simulink model "part3_3_b"  (R2017b)
settings: Solver=VariableStepAuto  StartTime=0.0  StopTime=0.1  RelTol=1e-3
libraries: simulink x1
settings Model: Creator=think  LastModifiedBy=think

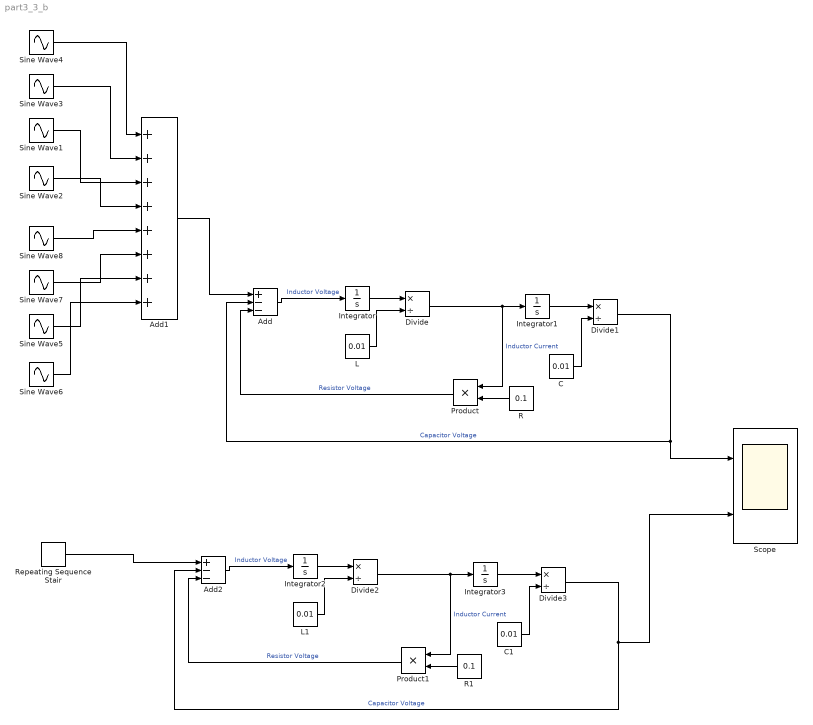
== system part3_3_b ==
  Add : Sum  Inputs=+--
  Add1 : Sum  Inputs=++++++++
  Add2 : Sum  Inputs=+--
  C : Constant  Value=0.01
  C1 : Constant  Value=0.01
  Divide{,1..3} (4 alike) : Product  Inputs=*/
  Integrator{,1..3} (4 alike) : Integrator
  L : Constant  Value=0.01
  L1 : Constant  Value=0.01
  Product : Product
  Product1 : Product
  R : Constant  Value=0.1
  R1 : Constant  Value=0.1
  Repeating Sequence Stair : simulink/Sources/Repeating Sequence Stair  OutValues=[1 -1]  tsamp=1/64  OutMin=[]  OutMax=[]  OutDataTypeStr=double  OutputDataTypeScalingMode=double  OutDataType=fixdt(0,8)  ConRadixGroup=Best Precision: Vector-wise  OutScaling=2^-12
  Scope : Scope  NumInputPorts=2
  Sine Wave1 : Sin  Amplitude=(4/pi)/5  Frequency=2*pi*32*5  SampleTime=0
  Sine Wave2 : Sin  Amplitude=(4/pi)/7  Frequency=2*pi*32*7  SampleTime=0
  Sine Wave3 : Sin  Amplitude=(4/pi)/3  Frequency=(2*pi*32)*3  SampleTime=0
  Sine Wave4 : Sin  Amplitude=4/pi  Frequency=2*pi*32  SampleTime=0
  Sine Wave5 : Sin  Amplitude=(4/pi)/13  Frequency=2*pi*32*13  SampleTime=0
  Sine Wave6 : Sin  Amplitude=(4/pi)/15  Frequency=2*pi*32*15  SampleTime=0
  Sine Wave7 : Sin  Amplitude=(4/pi)/11  Frequency=(2*pi*32)*11  SampleTime=0
  Sine Wave8 : Sin  Amplitude=4/pi/9  Frequency=2*pi*32*9  SampleTime=0
  wires:
  C/1 -> Divide1/2
  Integrator/1 -> Divide/1
  Integrator1/1 -> Divide1/1
  Divide/1 -> Integrator1/1, Product/1  "Inductor Current"
  Add/1 -> Integrator/1  "Inductor Voltage"
  Product/1 -> Add/3  "Resistor Voltage"
  L/1 -> Divide/2
  R/1 -> Product/2
  Divide1/1 -> Add/2, Scope/1  "Capacitor Voltage"
  Sine Wave2/1 -> Add1/4
  Sine Wave1/1 -> Add1/3
  Sine Wave4/1 -> Add1/1
  Sine Wave3/1 -> Add1/2
  Add1/1 -> Add/1
  Integrator3/1 -> Divide3/1
  Add2/1 -> Integrator2/1  "Inductor Voltage"
  Divide2/1 -> Integrator3/1, Product1/1  "Inductor Current"
  C1/1 -> Divide3/2
  Product1/1 -> Add2/3  "Resistor Voltage"
  R1/1 -> Product1/2
  Divide3/1 -> Scope/2, Add2/2  "Capacitor Voltage"
  L1/1 -> Divide2/2
  Integrator2/1 -> Divide2/1
  Repeating Sequence Stair/1 -> Add2/1
  Sine Wave8/1 -> Add1/5
  Sine Wave7/1 -> Add1/6
  Sine Wave5/1 -> Add1/7
  Sine Wave6/1 -> Add1/8
